simulink model "four_reaction_wheel_controller"  (R2026a)
settings: Solver=VariableStepAuto
undefined symbols (not defined in the file): Kd, Kp
settings Model: Creator=taizo  LastModifiedBy=aditi

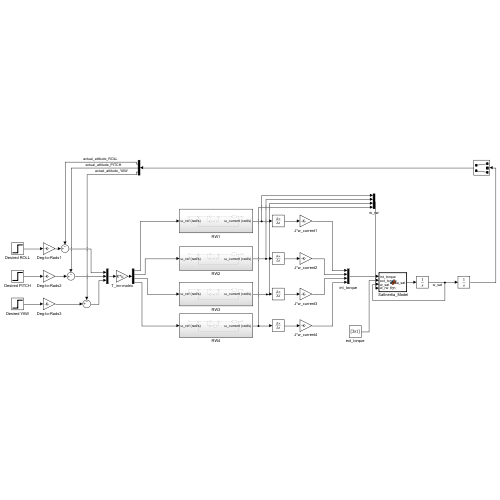
[thumbnail: Simulink's stored preview of the top-level diagram]
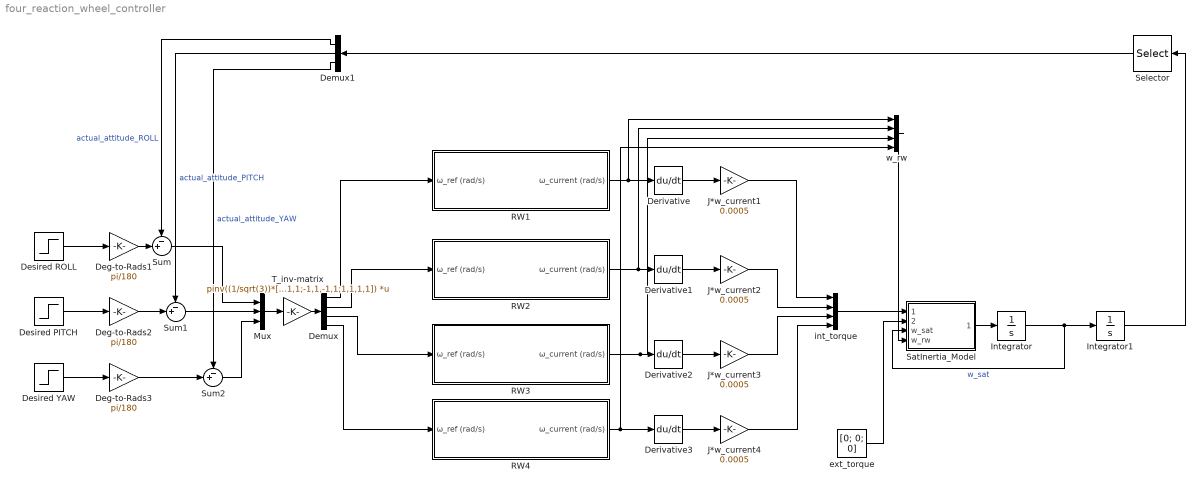
== system four_reaction_wheel_controller ==
  " SatInertia_Model" : MATLAB Function  TreatAsAtomicUnit=on
  Deg-to-Rads1 : Gain  Gain=pi/180
  Deg-to-Rads2 : Gain  Gain=pi/180
  Deg-to-Rads3 : Gain  Gain=pi/180
  Demux : Demux
  Demux1 : Demux  Outputs=3
  Derivative{,1..3} (4 alike) : Derivative
  Desired PITCH : Step  SampleTime=0
  Desired ROLL : Step  SampleTime=0
  Desired YAW : Step  SampleTime=0
  Integrator : Integrator
  Integrator1 : Integrator
  J*w_current{1..4} (4 alike) : Gain  Gain=0.0005
  Mux : Mux  Inputs=3
  RW1 : Subsystem
  RW2 : Subsystem
  RW3 : Subsystem
  RW4 : Subsystem
  Selector : Selector  InputPortWidth=3  IndexOptions=Index vector (dialog)  Indices=[1 3]  OutputSizes=1
  Sum : Sum  Inputs=-+|
  Sum1 : Sum  Inputs=-+|
  Sum2 : Sum  Inputs=-+|
  T_inv-matrix : Gain  Gain=pinv((1/sqrt(3))*[1,-1,-1,1;-1,1,-1,1;1,1,1,1])  Multiplication=Matrix(K*u)
  ext_torque : Constant  Value=[0; 0; 0]
  int_torque : Mux
  w_rw : Mux
  wires:
  Desired ROLL/1 -> Deg-to-Rads1/1
  Desired PITCH/1 -> Deg-to-Rads2/1
  Desired YAW/1 -> Deg-to-Rads3/1
  Deg-to-Rads1/1 -> Sum/2
  Deg-to-Rads2/1 -> Sum1/2
  Deg-to-Rads3/1 -> Sum2/2
  Sum/1 -> Mux/1
  Sum1/1 -> Mux/2
  Sum2/1 -> Mux/3
  Mux/1 -> T_inv-matrix/1
  T_inv-matrix/1 -> Demux/1
  Demux/1 -> RW1/1(ω_ref (rad/s))
  Demux/2 -> RW2/1(ω_ref (rad/s))
  Demux/3 -> RW3/1(ω_ref (rad/s))
  Demux/4 -> RW4/1(ω_ref (rad/s))
  RW1/1(ω_current (rad/s)) -> w_rw/1, Derivative/1
  RW2/1(ω_current (rad/s)) -> w_rw/2, Derivative1/1
  RW3/1(ω_current (rad/s)) -> w_rw/3, Derivative2/1
  RW4/1(ω_current (rad/s)) -> w_rw/4, Derivative3/1
  Derivative/1 -> J*w_current1/1
  Derivative1/1 -> J*w_current2/1
  Derivative2/1 -> J*w_current3/1
  Derivative3/1 -> J*w_current4/1
  J*w_current1/1 -> int_torque/1
  J*w_current2/1 -> int_torque/2
  J*w_current3/1 -> int_torque/3
  J*w_current4/1 -> int_torque/4
  w_rw/1 -> " SatInertia_Model"/4(w_rw)
  int_torque/1 -> " SatInertia_Model"/1(int_torque)
  ext_torque/1 -> " SatInertia_Model"/2(ext_torque)
  " SatInertia_Model"/1(alpha_sat) -> Integrator/1
  Integrator/1 -> " SatInertia_Model"/3(w_sat), Integrator1/1  "w_sat"
  Integrator1/1 -> Selector/1
  Selector/1 -> Demux1/1
  Demux1/1 -> Sum/1  "actual_attitude_ROLL"
  Demux1/2 -> Sum1/1  "actual_attitude_PITCH"
  Demux1/3 -> Sum2/1  "actual_attitude_YAW"

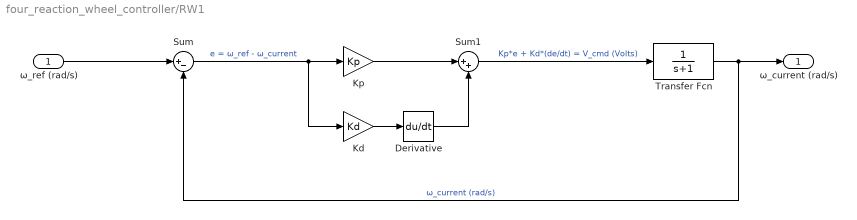
== system four_reaction_wheel_controller/RW1 ==
  ω_ref (rad/s) : Inport
  Derivative : Derivative
  Kd : Gain  Gain=Kd
  Kp : Gain  Gain=Kp
  Sum : Sum  Inputs=|+-
  Sum1 : Sum  Inputs=|++
  Transfer Fcn : TransferFcn  Denominator=[1 1]
  ω_current (rad/s) : Outport
  wires:
  ω_ref (rad/s)/1 -> Sum/1
  Kp/1 -> Sum1/1
  Sum1/1 -> Transfer Fcn/1  "Kp*e + Kd*(de/dt) = V_cmd (Volts)"
  Derivative/1 -> Sum1/2
  Sum/1 -> Kd/1, Kp/1  "e = ω_ref - ω_current"
  Kd/1 -> Derivative/1
  Transfer Fcn/1 -> ω_current (rad/s)/1, Sum/2  "ω_current (rad/s)"

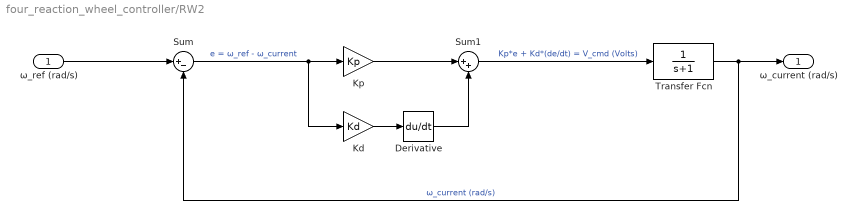
== system four_reaction_wheel_controller/RW2 ==
  ω_ref (rad/s) : Inport
  Derivative : Derivative
  Kd : Gain  Gain=Kd
  Kp : Gain  Gain=Kp
  Sum : Sum  Inputs=|+-
  Sum1 : Sum  Inputs=|++
  Transfer Fcn : TransferFcn  Denominator=[1 1]
  ω_current (rad/s) : Outport
  wires:
  ω_ref (rad/s)/1 -> Sum/1
  Kp/1 -> Sum1/1
  Sum1/1 -> Transfer Fcn/1  "Kp*e + Kd*(de/dt) = V_cmd (Volts)"
  Derivative/1 -> Sum1/2
  Sum/1 -> Kd/1, Kp/1  "e = ω_ref - ω_current"
  Kd/1 -> Derivative/1
  Transfer Fcn/1 -> ω_current (rad/s)/1, Sum/2  "ω_current (rad/s)"

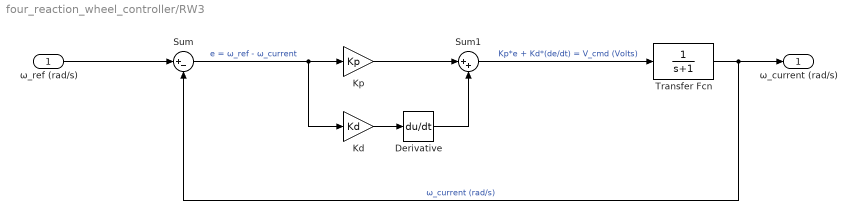
== system four_reaction_wheel_controller/RW3 ==
  ω_ref (rad/s) : Inport
  Derivative : Derivative
  Kd : Gain  Gain=Kd
  Kp : Gain  Gain=Kp
  Sum : Sum  Inputs=|+-
  Sum1 : Sum  Inputs=|++
  Transfer Fcn : TransferFcn  Denominator=[1 1]
  ω_current (rad/s) : Outport
  wires:
  ω_ref (rad/s)/1 -> Sum/1
  Kp/1 -> Sum1/1
  Sum1/1 -> Transfer Fcn/1  "Kp*e + Kd*(de/dt) = V_cmd (Volts)"
  Derivative/1 -> Sum1/2
  Sum/1 -> Kd/1, Kp/1  "e = ω_ref - ω_current"
  Kd/1 -> Derivative/1
  Transfer Fcn/1 -> ω_current (rad/s)/1, Sum/2  "ω_current (rad/s)"

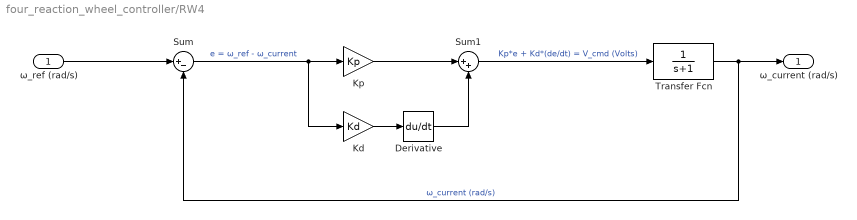
== system four_reaction_wheel_controller/RW4 ==
  ω_ref (rad/s) : Inport
  Derivative : Derivative
  Kd : Gain  Gain=Kd
  Kp : Gain  Gain=Kp
  Sum : Sum  Inputs=|+-
  Sum1 : Sum  Inputs=|++
  Transfer Fcn : TransferFcn  Denominator=[1 1]
  ω_current (rad/s) : Outport
  wires:
  ω_ref (rad/s)/1 -> Sum/1
  Kp/1 -> Sum1/1
  Sum1/1 -> Transfer Fcn/1  "Kp*e + Kd*(de/dt) = V_cmd (Volts)"
  Derivative/1 -> Sum1/2
  Sum/1 -> Kd/1, Kp/1  "e = ω_ref - ω_current"
  Kd/1 -> Derivative/1
  Transfer Fcn/1 -> ω_current (rad/s)/1, Sum/2  "ω_current (rad/s)"

== matlab function four_reaction_wheel_controller/ SatInertia_Model ==
  data: int_torque input; alpha_sat output; ext_torque input; w_sat input; w_rw input
function alpha_sat = fcn(int_torque, ext_torque, w_sat, w_rw)

    % Spacecraft inertia (kg·m²) - change to your values
    Jx = 0.05; 
    Jy = 0.05; 
    Jz = 0.1;
    J = diag([Jx, Jy, Jz]);

    % Wheel inertia (kg·m²)
    Jw = 0.0005;

    % Distribution matrix
    T = (1/sqrt(3)) * [1,-1,-1, 1;
                      -1, 1,-1, 1;
                       1, 1, 1, 1];

    % Wheel angular momentum in body frame
    H_rw = T * (Jw * w_rw);

    % Gyroscopic term
    gyro = cross(w_sat, J*w_sat + H_rw);

    % Angular acceleration
    alpha_sat = J \ (int_torque + ext_torque - gyro);

end
